simulink model "Sim47"  (R2019a)
settings: Solver=FixedStepAuto  StartTime=0.0  StopTime=10.0  FixedStep=0.0001  RelTol=1e-3
settings Model: Creator=fbleo  LastModifiedBy=fbleo

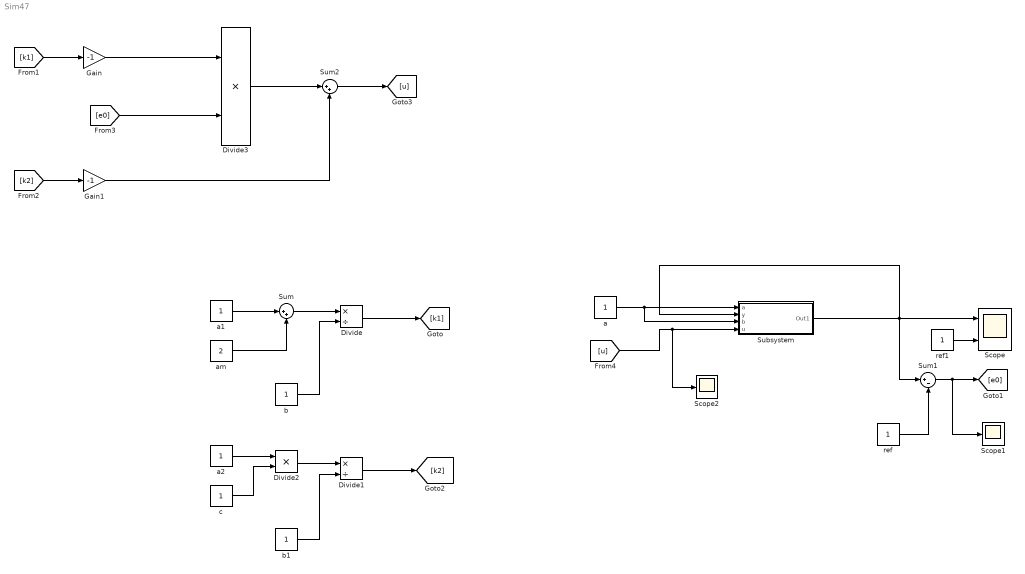
== system Sim47 ==
  Divide : Product  Inputs=*/
  Divide1 : Product  Inputs=*/
  Divide2 : Product  Inputs=**
  Divide3 : Product  Inputs=**
  Gain : Gain  Gain=-1
  Gain1 : Gain  Gain=-1
  Scope : Scope  NumInputPorts=2
  Scope1 : Scope
  Scope2 : Scope
  Subsystem : Subsystem
  Sum : Sum  Inputs=|++
  Sum1 : Sum  Inputs=|+-
  Sum2 : Sum  Inputs=|++
  a : Constant
  a1 : Constant
  a2 : Constant
  am : Constant  Value=2
  b : Constant
  b1 : Constant
  c : Constant
  ref : Constant
  ref1 : Constant
  wires:
  Divide/1 -> [k1]
  am/1 -> Sum/2
  a1/1 -> Sum/1
  b/1 -> Divide/2
  Subsystem/1(Out1) -> Subsystem/2(y), Scope/1, Sum1/1
  Sum/1 -> Divide/1
  a/1 -> Subsystem/3(b), Subsystem/1(a)
  ref/1 -> Sum1/2
  Sum1/1 -> Scope1/1, [e0]
  b1/1 -> Divide1/2
  a2/1 -> Divide2/1
  Divide2/1 -> Divide1/1
  Divide1/1 -> [k2]
  c/1 -> Divide2/2
  [k1] -> Gain/1
  [k2] -> Gain1/1
  Gain/1 -> Divide3/1
  [e0] -> Divide3/2
  [u] -> Scope2/1, Subsystem/4(u)
  Divide3/1 -> Sum2/1
  Gain1/1 -> Sum2/2
  Sum2/1 -> [u]
  ref1/1 -> Scope/2

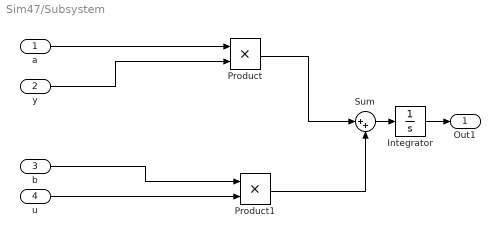
== system Sim47/Subsystem ==
  a : Inport
  y : Inport  Port=2
  b : Inport  Port=3
  u : Inport  Port=4
  Integrator : Integrator  InitialCondition=0.5
  Product : Product
  Product1 : Product
  Sum : Sum  Inputs=|++
  Out1 : Outport
  wires:
  a/1 -> Product/1
  y/1 -> Product/2
  Product/1 -> Sum/1
  u/1 -> Product1/2
  b/1 -> Product1/1
  Product1/1 -> Sum/2
  Sum/1 -> Integrator/1
  Integrator/1 -> Out1/1
